simulink subsystem "Simple_Spring_and_Damper_Suspension"  (R2025b)
settings: Solver=VariableStepAuto  StartTime=0.0  StopTime=10.0  RelTol=1e-3
undefined symbols (not defined in the file): MotoFrntSuspDamp, MotoFrntSuspEqlbrmLngth, MotoFrntSuspStf
settings Model: Creator=The MathWorks, Inc.  LastModifiedBy=The MathWorks, Inc.
settings RTWCC: GPUComputeCapability=3.5

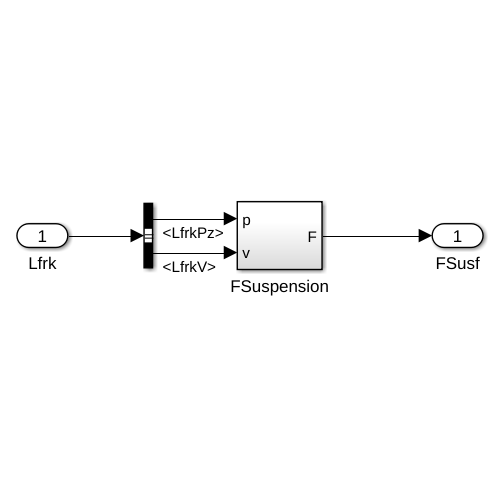
[thumbnail: Simulink's stored preview of the top-level diagram]
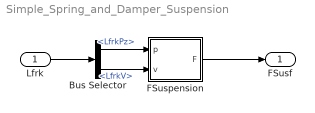
== system Simple_Spring_and_Damper_Suspension ==
  Lfrk : Inport
  Bus Selector : BusSelector  OutputSignals=LfrkPz,LfrkV
  FSuspension : Subsystem
  FSusf : Outport
  wires:
  Bus Selector/2 -> FSuspension/2(v)  "<LfrkV>"
  Bus Selector/1 -> FSuspension/1(p)  "<LfrkPz>"
  Lfrk/1 -> Bus Selector/1
  FSuspension/1(F) -> FSusf/1

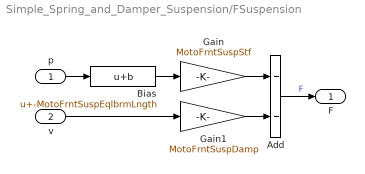
== system Simple_Spring_and_Damper_Suspension/FSuspension ==
  p : Inport
  v : Inport  Port=2
  Add : Sum  Inputs=--
  Bias : Bias  Bias=-MotoFrntSuspEqlbrmLngth  SaturateOnIntegerOverflow=off
  Gain : Gain  Gain=MotoFrntSuspStf
  Gain1 : Gain  Gain=MotoFrntSuspDamp
  F : Outport
  wires:
  p/1 -> Bias/1
  v/1 -> Gain1/1
  Gain1/1 -> Add/2
  Gain/1 -> Add/1
  Add/1 -> F/1  "F"
  Bias/1 -> Gain/1
